simulink model "nlfm"  (R2023b)
settings: Solver=FixedStepAuto  StartTime=0.0  StopTime=10.0  FixedStep=5.3333333333333331e-09  RelTol=1e-3
undefined symbols (not defined in the file): jsin
libraries: hdlsllib x2, simulink x1
settings Model: Creator=mori  LastModifiedBy=mori
settings DataIOCC: SaveOutput=off  SaveTime=off

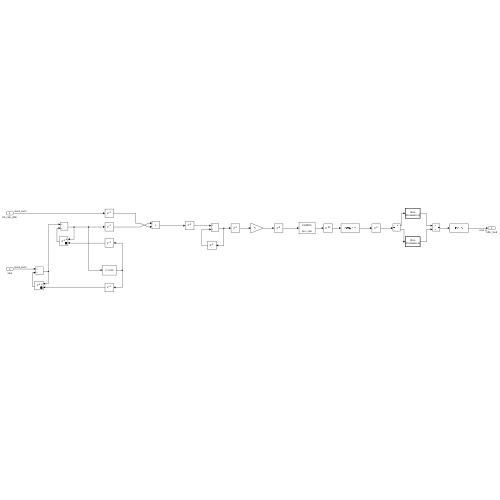
[thumbnail: Simulink's stored preview of the top-level diagram]
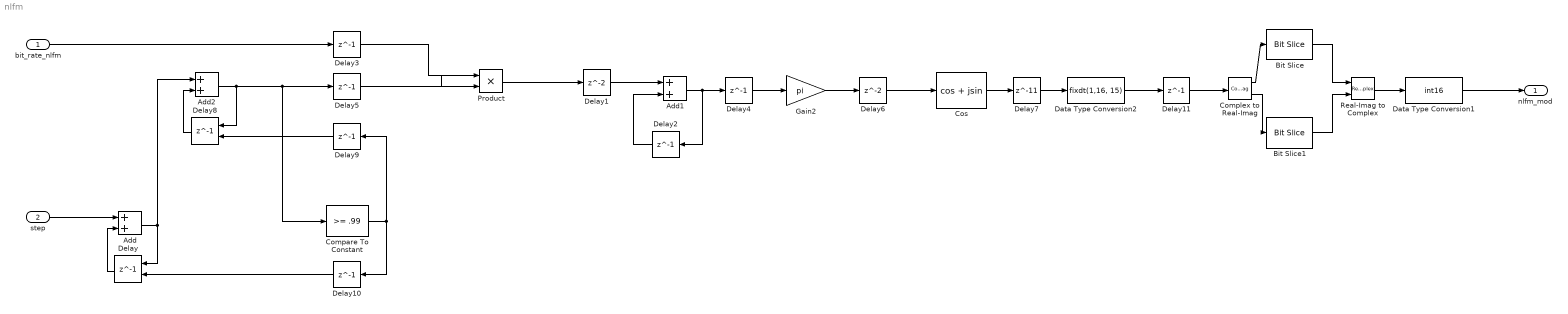
== system nlfm ==
  bit_rate_nlfm : Inport  OutDataTypeStr=fixdt(1,24,23)  PortDimensions=1  SampleTime=[5.3333333333333331e-09,0]
  step : Inport  Port=2  OutDataTypeStr=fixdt(1,24,23)  PortDimensions=1  SampleTime=[5.3333333333333331e-09,0]
  Add : Sum  OutDataTypeStr=fixdt(1,24, 23)
  Add1 : Sum  OutDataTypeStr=Inherit: Same as first input
  Add2 : Sum  OutDataTypeStr=fixdt(1,24, 23)  SaturateOnIntegerOverflow=on
  Bit Slice : hdlsllib/Logic and Bit Operations/Bit Slice  lidx=15  ridx=0
  Bit Slice1 : hdlsllib/Logic and Bit Operations/Bit Slice  lidx=15  ridx=0
  Compare To Constant : simulink/Logic and Bit Operations/Compare To Constant  relop=>=  const=.99  OutDataTypeStr=boolean
  Complex to Real-Imag : ComplexToRealImag
  Cos : Trigonometry  Operator=cos + jsin  ApproximationMethod=CORDIC
  Data Type Conversion1 : DataTypeConversion  OutDataTypeStr=int16  SaturateOnIntegerOverflow=off  RndMeth=Floor
  Data Type Conversion2 : DataTypeConversion  OutDataTypeStr=fixdt(1,16, 15)  RndMeth=Nearest
  Delay : Delay  DelayLength=1  ExternalReset=Level
      settings: InputPortMap=u0,r5
  Delay1 : Delay
  Delay{3,5,9..10} (4 alike) : Delay  DelayLength=1  SampleTime=1/187.5e6
  Delay11 : Delay  DelayLength=1
  Delay2 : Delay  DelayLength=1
  Delay4 : Delay  DelayLength=1
  Delay6 : Delay
  Delay7 : Delay  DelayLength=11
  Delay8 : Delay  DelayLength=1  InitialCondition=-1  ExternalReset=Level
      settings: InputPortMap=u0,r5
  Gain2 : Gain  Gain=pi  OutDataTypeStr=fixdt(1,24,20)
  Product : Product  OutDataTypeStr=Inherit: Same as first input
  Real-Imag to Complex : RealImagToComplex
  nlfm_mod : Outport  OutDataTypeStr=int16  PortDimensions=1  SampleTime=[5.3333333333333331e-09,0]
      settings: SignalType=complex
  wires:
  Delay2/1 -> Add1/2
  Delay9/1 -> Delay8/2
  Delay6/1 -> Cos/1
  Cos/1 -> Delay7/1
  Delay3/1 -> Product/2
  Delay8/1 -> Add2/2
  Data Type Conversion2/1 -> Delay11/1
  Add1/1 -> Delay4/1, Delay2/1
  Delay1/1 -> Add1/1
  Delay7/1 -> Data Type Conversion2/1
  Delay5/1 -> Product/1
  Product/1 -> Delay1/1
  Add2/1 -> Compare To Constant/1, Delay5/1, Delay8/1
  Complex to Real-Imag/2 -> Bit Slice1/1
  Complex to Real-Imag/1 -> Bit Slice/1
  Delay10/1 -> Delay/2
  Compare To Constant/1 -> Delay10/1, Delay9/1
  Delay11/1 -> Complex to Real-Imag/1
  Delay/1 -> Add/2
  Bit Slice1/1 -> Real-Imag to Complex/2
  step/1 -> Add/1
  Gain2/1 -> Delay6/1
  Bit Slice/1 -> Real-Imag to Complex/1
  Add/1 -> Delay/1, Add2/1
  Real-Imag to Complex/1 -> Data Type Conversion1/1
  Delay4/1 -> Gain2/1
  bit_rate_nlfm/1 -> Delay3/1
  Data Type Conversion1/1 -> nlfm_mod/1
